simulink model "sim_sistema_4"  (Simulink 7.5)
settings: Solver=ode45  StartTime=0.0  StopTime=25  FixedStep=1e-4  RelTol=1e-3
values from neighbouring files (symbols this model uses):
  A = [0 1 0 0;20.601 0 0 0;0 0 0 1;-0.4905 0 0 0]    [sistema_4_observador.m]
  B = [0 -1 0 0.5]'    [sistema_4_observador.m]
  C = [0 0 1 0]    [sistema_4_observador.m]
  K = K(1:end-1)    [sistema_4_observador.m]
  Ke = phi*inv(CA)*col    [sistema_4_observador.m]
  KI = K(end)    [sistema_4_observador.m]
settings Model: Creator=taniel.franklin  LastModifiedBy=taniel.franklin

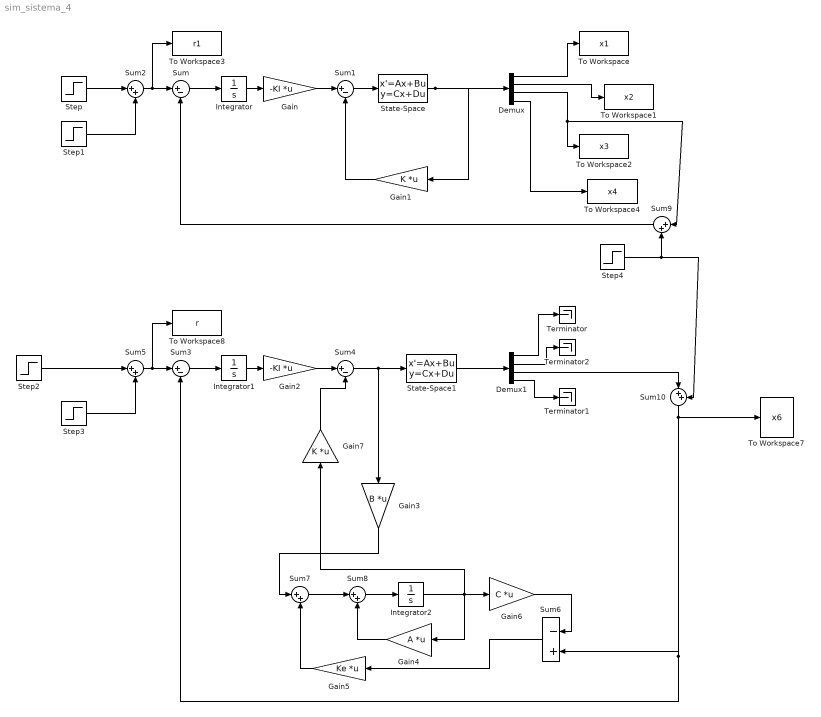
== system sim_sistema_4 ==
  Demux : Demux
  Demux1 : Demux
  Gain : Gain  Gain=-KI  Multiplication=Matrix(K*u)  ParameterDataType=fixdt(1, 16)  ParameterScaling=2^0  OutDataType=fixdt(1, 16)  OutScaling=2^0
  Gain1 : Gain  Gain=K  Multiplication=Matrix(K*u)  ParameterDataType=fixdt(1, 16)  ParameterScaling=2^0  OutDataType=fixdt(1, 16)  OutScaling=2^0
  Gain2 : Gain  Gain=-KI  Multiplication=Matrix(K*u)  ParameterDataType=fixdt(1, 16)  ParameterScaling=2^0  OutDataType=fixdt(1, 16)  OutScaling=2^0
  Gain3 : Gain  Gain=B  Multiplication=Matrix(K*u)  ParameterDataType=fixdt(1, 16)  ParameterScaling=2^0  OutDataType=fixdt(1, 16)  OutScaling=2^0
  Gain4 : Gain  Gain=A  Multiplication=Matrix(K*u)  ParameterDataType=fixdt(1, 16)  ParameterScaling=2^0  OutDataType=fixdt(1, 16)  OutScaling=2^0
  Gain5 : Gain  Gain=Ke  Multiplication=Matrix(K*u)  ParameterDataType=fixdt(1, 16)  ParameterScaling=2^0  OutDataType=fixdt(1, 16)  OutScaling=2^0
  Gain6 : Gain  Gain=C  Multiplication=Matrix(K*u)  ParameterDataType=fixdt(1, 16)  ParameterScaling=2^0  OutDataType=fixdt(1, 16)  OutScaling=2^0
  Gain7 : Gain  Gain=K  Multiplication=Matrix(K*u)  ParameterDataType=fixdt(1, 16)  ParameterScaling=2^0  OutDataType=fixdt(1, 16)  OutScaling=2^0
  Integrator : Integrator
  Integrator1 : Integrator
  Integrator2 : Integrator
  State-Space : StateSpace  A=A  B=B  C=eye(4)  D=[0;0;0;0]
  State-Space1 : StateSpace  A=A  B=B  C=eye(4)  D=[0;0;0;0]
  Step : Step  Time=0.1  SampleTime=0
  Step1 : Step  Time=8  SampleTime=0
  Step2 : Step  Time=0.1  SampleTime=0
  Step3 : Step  Time=8  SampleTime=0
  Step4 : Step  Time=15  After=0.1  SampleTime=0
  Sum{,1,3..4} (4 alike) : Sum  Inputs=|+-  OutDataType=fixdt(1, 16)  OutScaling=2^0
  Sum{2,5,7..10} (6 alike) : Sum  Inputs=|++  OutDataType=fixdt(1, 16)  OutScaling=2^0
  Sum6 : Sum  Inputs=|-+  OutDataType=fixdt(1, 16)  OutScaling=2^0
  Terminator : Terminator
  Terminator1 : Terminator
  Terminator2 : Terminator
  To Workspace : ToWorkspace  VariableName=x1  SampleTime=-1  SaveFormat=Structure With Time
  To Workspace1 : ToWorkspace  VariableName=x2  SampleTime=-1  SaveFormat=Structure With Time
  To Workspace2 : ToWorkspace  VariableName=x3  SampleTime=-1  SaveFormat=Structure With Time
  To Workspace3 : ToWorkspace  VariableName=r1  SampleTime=-1  SaveFormat=Structure With Time
  To Workspace4 : ToWorkspace  VariableName=x4  SampleTime=-1  SaveFormat=Structure With Time
  To Workspace7 : ToWorkspace  VariableName=x6  SampleTime=-1  SaveFormat=Structure With Time
  To Workspace8 : ToWorkspace  VariableName=r  SampleTime=-1  SaveFormat=Structure With Time
  wires:
  State-Space/1 -> Demux/1, Gain1/1
  Demux/2 -> To Workspace1/1
  Demux/3 -> To Workspace2/1, Sum9/1
  Sum/1 -> Integrator/1
  Sum1/1 -> State-Space/1
  Step/1 -> Sum2/1
  Step1/1 -> Sum2/2
  Sum2/1 -> Sum/1, To Workspace3/1
  Demux/1 -> To Workspace/1
  Gain1/1 -> Sum1/2
  Demux/4 -> To Workspace4/1
  Integrator/1 -> Gain/1
  Gain/1 -> Sum1/1
  State-Space1/1 -> Demux1/1
  Sum3/1 -> Integrator1/1
  Sum4/1 -> State-Space1/1, Gain3/1
  Step3/1 -> Sum5/2
  Sum5/1 -> To Workspace8/1, Sum3/1
  Integrator1/1 -> Gain2/1
  Gain2/1 -> Sum4/1
  Sum6/1 -> Gain5/1
  Gain5/1 -> Sum7/2
  Gain3/1 -> Sum7/1
  Sum8/1 -> Integrator2/1
  Sum7/1 -> Sum8/1
  Integrator2/1 -> Gain4/1, Gain6/1, Gain7/1
  Gain4/1 -> Sum8/2
  Gain6/1 -> Sum6/1
  Gain7/1 -> Sum4/2
  Demux1/1 -> Terminator/1
  Demux1/4 -> Terminator1/1
  Demux1/2 -> Terminator2/1
  Step2/1 -> Sum5/1
  Sum9/1 -> Sum/2
  Step4/1 -> Sum9/2, Sum10/2
  Demux1/3 -> Sum10/1
  Sum10/1 -> To Workspace7/1, Sum6/2, Sum3/2
